simulink model "Verification_Component_Primitive_replacement"  (R2012b)
settings: Solver=FixedStepDiscrete  StartTime=0.0  StopTime=10.0  FixedStep=0.1  RelTol=1e-3
libraries: sldvlib x15, simulink x1
settings Model: sldv_blockreplacement_configurable_lib=Verification_Component_Primitive_rt_lib  Creator=Kerianne  LastModifiedBy=Kerianne
settings DataIOCC: SaveFormat=Structure
settings OptimizationCC: InlineParams=on
settings DebuggingCC: ArtificialAlgebraicLoopMsg=none

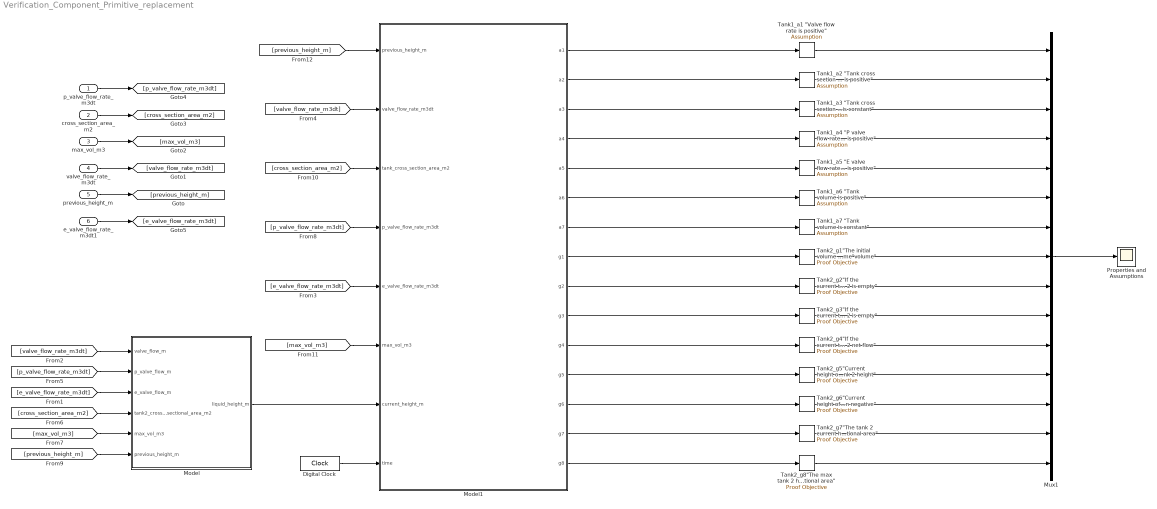
== system Verification_Component_Primitive_replacement ==
  p_valve_flow_rate_m3dt : Inport  OutDataTypeStr=double
  cross_section_area_m2 : Inport  Port=2  OutDataTypeStr=double
  max_vol_m3 : Inport  Port=3  OutDataTypeStr=double
  valve_flow_rate_m3dt : Inport  Port=4  OutDataTypeStr=double
  previous_height_m : Inport  Port=5  OutDataTypeStr=double
  e_valve_flow_rate_m3dt1 : Inport  Port=6  OutDataTypeStr=double
  Digital Clock : DigitalClock  SampleTime=0.1
  Model : Subsystem  TreatAsAtomicUnit=on  mask(Sldv ModelReference(Model name:Tank2_Primitives) Replacement){ModelName=Tank2_Primitives, ParameterArgumentNames=, ParameterArgumentValues=, SimulationMode=Normal}
      mask help: Replacement for the Model Reference block that references the model Tank2_Primitives. If Model arguments are specified on the Model Reference block, then they will appear in the mask parameters.
  Model1 : Subsystem  TreatAsAtomicUnit=on  mask(Sldv ModelReference(Model name:Properties_Tank2_Primitives) Replacement){ModelName=Properties_Tank2_Primitives, ParameterArgumentNames=, ParameterArgumentValues=, SimulationMode=Normal}
      mask help: Replacement for the Model Reference block that references the model Properties_Tank2_Primitives. If Model arguments are specified on the Model Reference block, then they will appear in the mask parameters.
  Mux1 : Mux  Inputs=15
  Properties and Assumptions : Scope
      settings: ShowLegends=on
  "Tank1_a1 \"Valve flow rate is positive\"" : sldvlib/Objectives and Constraints/Assumption  enabled=on  customAVTBlockType=Assumption  intervals=true  initial=off  dispValues=on  outEnabled=on
      settings: AttributesFormatString=%<intervals>
  "Tank1_a2 \"Tank cross section area is positive\"" : sldvlib/Objectives and Constraints/Assumption  enabled=on  customAVTBlockType=Assumption  intervals=true  initial=off  dispValues=on  outEnabled=on
      settings: AttributesFormatString=%<intervals>
  "Tank1_a3 \"Tank cross section area is constant\"" : sldvlib/Objectives and Constraints/Assumption  enabled=on  customAVTBlockType=Assumption  intervals=true  initial=off  dispValues=on  outEnabled=on
      settings: AttributesFormatString=%<intervals>
  "Tank1_a4 \"P valve flow rate is positive\"" : sldvlib/Objectives and Constraints/Assumption  enabled=on  customAVTBlockType=Assumption  intervals=true  initial=off  dispValues=on  outEnabled=on
      settings: AttributesFormatString=%<intervals>
  "Tank1_a5 \"E valve flow rate is positive\"" : sldvlib/Objectives and Constraints/Assumption  enabled=on  customAVTBlockType=Assumption  intervals=true  initial=off  dispValues=on  outEnabled=on
      settings: AttributesFormatString=%<intervals>
  "Tank1_a6 \"Tank volume is positive\"" : sldvlib/Objectives and Constraints/Assumption  enabled=on  customAVTBlockType=Assumption  intervals=true  initial=off  dispValues=on  outEnabled=on
      settings: AttributesFormatString=%<intervals>
  "Tank1_a7 \"Tank volume is constant\"" : sldvlib/Objectives and Constraints/Assumption  enabled=on  customAVTBlockType=Assumption  intervals=true  initial=off  dispValues=on  outEnabled=on
      settings: AttributesFormatString=%<intervals>
  "Tank2_g1\"The initial volume of tank 2 should be equivalent to the specified initial tank 2 volume\"volume\" " : sldvlib/Objectives and Constraints/Proof Objective  enabled=on  customAVTBlockType=Proof Objective  intervals=true  dispValues=on  outEnabled=on  enableStopSim=off
      settings: AttributesFormatString=%<intervals>
  "Tank2_g2\"If the current tank 2 volume plus the tank 2 net flow is less than the tank 2 minimum volume then tank 2 is empty\" " : sldvlib/Objectives and Constraints/Proof Objective  enabled=on  customAVTBlockType=Proof Objective  intervals=true  dispValues=on  outEnabled=on  enableStopSim=off
      settings: AttributesFormatString=%<intervals>
  "Tank2_g3\"If the current tank 2 volume plus the tank 2 net flow is less than the tank 2 minimum volume then tank 2 is empty\"" : sldvlib/Objectives and Constraints/Proof Objective  enabled=on  customAVTBlockType=Proof Objective  intervals=true  dispValues=on  outEnabled=on  enableStopSim=off
      settings: AttributesFormatString=%<intervals>
  "Tank2_g4\"If the current tank 2 volume plus the tank 2 net flow is greater than empty and less than the tank 2 maximum volume then the tank 2 volume changes by the tank 2 net flow\"" : sldvlib/Objectives and Constraints/Proof Objective  enabled=on  customAVTBlockType=Proof Objective  intervals=true  dispValues=on  outEnabled=on  enableStopSim=off
      settings: AttributesFormatString=%<intervals>
  "Tank2_g5\"Current height of tank 2 is equal or less than the max tank 2 height\"" : sldvlib/Objectives and Constraints/Proof Objective  enabled=on  customAVTBlockType=Proof Objective  intervals=true  dispValues=on  outEnabled=on  enableStopSim=off
      settings: AttributesFormatString=%<intervals>
  "Tank2_g6\"Current height of tank 2 is non negative\"" : sldvlib/Objectives and Constraints/Proof Objective  enabled=on  customAVTBlockType=Proof Objective  intervals=true  dispValues=on  outEnabled=on  enableStopSim=off
      settings: AttributesFormatString=%<intervals>
  "Tank2_g7\"The tank 2 current height is equal to the tank 2 current volume divided by the tank 2 cross sectional area\" " : sldvlib/Objectives and Constraints/Proof Objective  enabled=on  customAVTBlockType=Proof Objective  intervals=true  dispValues=on  outEnabled=on  enableStopSim=off
      settings: AttributesFormatString=%<intervals>
  "Tank2_g8\"The max tank 2 height is equal to the max tank 2 volume divided by tank 2 cross sectional area\"" : sldvlib/Objectives and Constraints/Proof Objective  enabled=on  customAVTBlockType=Proof Objective  intervals=true  dispValues=on  outEnabled=on  enableStopSim=off
      settings: AttributesFormatString=%<intervals>
  wires:
  Model/1(liquid_height_m) -> Model1/7(current_height_m)
  Mux1/1 -> Properties and Assumptions/1
  previous_height_m/1 -> [previous_height_m]
  valve_flow_rate_m3dt/1 -> [valve_flow_rate_m3dt]
  max_vol_m3/1 -> [max_vol_m3]
  p_valve_flow_rate_m3dt/1 -> [p_valve_flow_rate_m3dt]
  cross_section_area_m2/1 -> [cross_section_area_m2]
  Digital Clock/1 -> Model1/8(time)
  e_valve_flow_rate_m3dt1/1 -> [e_valve_flow_rate_m3dt]
  [valve_flow_rate_m3dt] -> Model/1(valve_flow_m)
  [p_valve_flow_rate_m3dt] -> Model/2(p_valve_flow_m)
  [e_valve_flow_rate_m3dt] -> Model/3(e_valve_flow_m)
  [cross_section_area_m2] -> Model/4(tank2_cross_sectional_area_m2)
  [max_vol_m3] -> Model/5(max_vol_m3)
  [previous_height_m] -> Model/6(previous_height_m)
  [previous_height_m] -> Model1/1(previous_height_m)
  [valve_flow_rate_m3dt] -> Model1/2(valve_flow_rate_m3dt)
  [cross_section_area_m2] -> Model1/3(tank_cross_section_area_m2)
  [p_valve_flow_rate_m3dt] -> Model1/4(p_valve_flow_rate_m3dt)
  [e_valve_flow_rate_m3dt] -> Model1/5(e_valve_flow_rate_m3dt)
  [max_vol_m3] -> Model1/6(max_vol_m3)
  Model1/7(a7) -> "Tank1_a7 \"Tank volume is constant\""/1
  Model1/6(a6) -> "Tank1_a6 \"Tank volume is positive\""/1
  Model1/5(a5) -> "Tank1_a5 \"E valve flow rate is positive\""/1
  Model1/4(a4) -> "Tank1_a4 \"P valve flow rate is positive\""/1
  Model1/3(a3) -> "Tank1_a3 \"Tank cross section area is constant\""/1
  Model1/2(a2) -> "Tank1_a2 \"Tank cross section area is positive\""/1
  Model1/1(a1) -> "Tank1_a1 \"Valve flow rate is positive\""/1
  "Tank1_a1 \"Valve flow rate is positive\""/1 -> Mux1/1
  "Tank1_a2 \"Tank cross section area is positive\""/1 -> Mux1/2
  "Tank1_a3 \"Tank cross section area is constant\""/1 -> Mux1/3
  "Tank1_a4 \"P valve flow rate is positive\""/1 -> Mux1/4
  "Tank1_a5 \"E valve flow rate is positive\""/1 -> Mux1/5
  "Tank1_a6 \"Tank volume is positive\""/1 -> Mux1/6
  "Tank1_a7 \"Tank volume is constant\""/1 -> Mux1/7
  Model1/8(g1) -> "Tank2_g1\"The initial volume of tank 2 should be equivalent to the specified initial tank 2 volume\"volume\" "/1
  Model1/9(g2) -> "Tank2_g2\"If the current tank 2 volume plus the tank 2 net flow is less than the tank 2 minimum volume then tank 2 is empty\" "/1
  Model1/10(g3) -> "Tank2_g3\"If the current tank 2 volume plus the tank 2 net flow is less than the tank 2 minimum volume then tank 2 is empty\""/1
  Model1/11(g4) -> "Tank2_g4\"If the current tank 2 volume plus the tank 2 net flow is greater than empty and less than the tank 2 maximum volume then the tank 2 volume changes by the tank 2 net flow\""/1
  Model1/12(g5) -> "Tank2_g5\"Current height of tank 2 is equal or less than the max tank 2 height\""/1
  Model1/13(g6) -> "Tank2_g6\"Current height of tank 2 is non negative\""/1
  Model1/14(g7) -> "Tank2_g7\"The tank 2 current height is equal to the tank 2 current volume divided by the tank 2 cross sectional area\" "/1
  Model1/15(g8) -> "Tank2_g8\"The max tank 2 height is equal to the max tank 2 volume divided by tank 2 cross sectional area\""/1
  "Tank2_g1\"The initial volume of tank 2 should be equivalent to the specified initial tank 2 volume\"volume\" "/1 -> Mux1/8
  "Tank2_g2\"If the current tank 2 volume plus the tank 2 net flow is less than the tank 2 minimum volume then tank 2 is empty\" "/1 -> Mux1/9
  "Tank2_g3\"If the current tank 2 volume plus the tank 2 net flow is less than the tank 2 minimum volume then tank 2 is empty\""/1 -> Mux1/10
  "Tank2_g4\"If the current tank 2 volume plus the tank 2 net flow is greater than empty and less than the tank 2 maximum volume then the tank 2 volume changes by the tank 2 net flow\""/1 -> Mux1/11
  "Tank2_g5\"Current height of tank 2 is equal or less than the max tank 2 height\""/1 -> Mux1/12
  "Tank2_g6\"Current height of tank 2 is non negative\""/1 -> Mux1/13
  "Tank2_g7\"The tank 2 current height is equal to the tank 2 current volume divided by the tank 2 cross sectional area\" "/1 -> Mux1/14
  "Tank2_g8\"The max tank 2 height is equal to the max tank 2 volume divided by tank 2 cross sectional area\""/1 -> Mux1/15

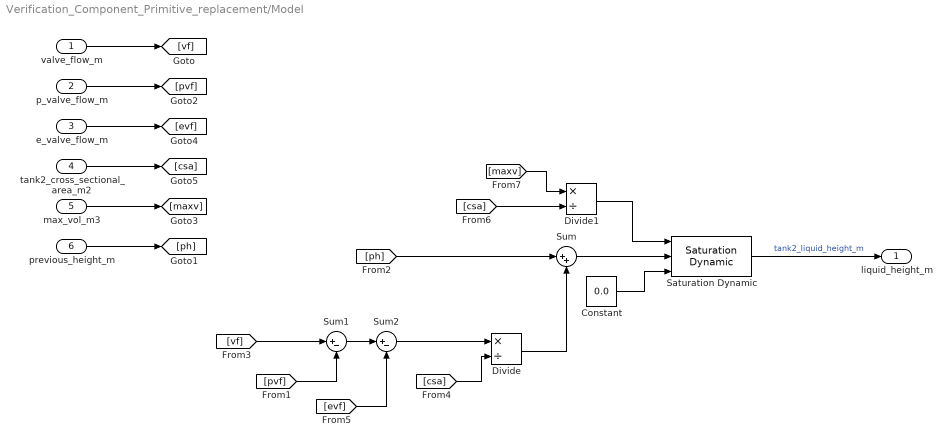
== system Verification_Component_Primitive_replacement/Model ==
  valve_flow_m : Inport  OutDataTypeStr=double  PortDimensions=1  SampleTime=[0.10000000000000001,0]
  p_valve_flow_m : Inport  Port=2  OutDataTypeStr=double  PortDimensions=1  SampleTime=[0.10000000000000001,0]
  e_valve_flow_m : Inport  Port=3  OutDataTypeStr=double  PortDimensions=1  SampleTime=[0.10000000000000001,0]
  tank2_cross_sectional_area_m2 : Inport  Port=4  OutDataTypeStr=double  PortDimensions=1  SampleTime=[0.10000000000000001,0]
  max_vol_m3 : Inport  Port=5  OutDataTypeStr=double  PortDimensions=1  SampleTime=[0.10000000000000001,0]
  previous_height_m : Inport  Port=6  OutDataTypeStr=double  PortDimensions=1  SampleTime=[0.10000000000000001,0]
  Constant : Constant  Value=0.0
  Divide : Product  Inputs=*/
  Divide1 : Product  Inputs=*/
  Saturation Dynamic : simulink/Discontinuities/Saturation Dynamic  OutMin=[]  OutMax=[]  OutDataTypeStr=Inherit: Same as second input  OutDataType=fixdt(1, 16)  OutScaling=2^-10  DoSatur=off
  Sum : Sum  Inputs=|++
  Sum1 : Sum  Inputs=|+-
  Sum2 : Sum  Inputs=|+-
  liquid_height_m : Outport  OutDataTypeStr=double  PortDimensions=1  SampleTime=[0.10000000000000001,0]
  wires:
  [evf] -> Sum2/2
  valve_flow_m/1 -> [vf]
  p_valve_flow_m/1 -> [pvf]
  Divide/1 -> Sum/2
  [csa] -> Divide/2
  [ph] -> Sum/1
  tank2_cross_sectional_area_m2/1 -> [csa]
  [vf] -> Sum1/1
  e_valve_flow_m/1 -> [evf]
  Sum2/1 -> Divide/1
  [pvf] -> Sum1/2
  Sum1/1 -> Sum2/1
  max_vol_m3/1 -> [maxv]
  Divide1/1 -> Saturation Dynamic/1
  Sum/1 -> Saturation Dynamic/2
  Constant/1 -> Saturation Dynamic/3
  [csa] -> Divide1/2
  [maxv] -> Divide1/1
  Saturation Dynamic/1 -> liquid_height_m/1  "tank2_liquid_height_m"
  previous_height_m/1 -> [ph]

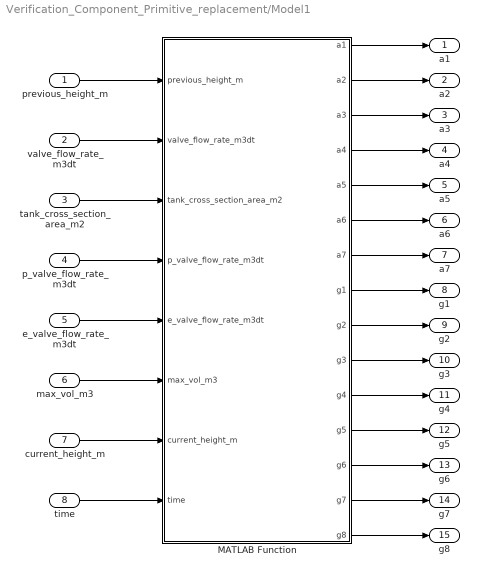
== system Verification_Component_Primitive_replacement/Model1 ==
  previous_height_m : Inport  OutDataTypeStr=double  PortDimensions=1  SampleTime=[0.10000000000000001,0]
  valve_flow_rate_m3dt : Inport  Port=2  OutDataTypeStr=double  PortDimensions=1  SampleTime=[0.10000000000000001,0]
  tank_cross_section_area_m2 : Inport  Port=3  OutDataTypeStr=double  PortDimensions=1  SampleTime=[0.10000000000000001,0]
  p_valve_flow_rate_m3dt : Inport  Port=4  OutDataTypeStr=double  PortDimensions=1  SampleTime=[0.10000000000000001,0]
  e_valve_flow_rate_m3dt : Inport  Port=5  OutDataTypeStr=double  PortDimensions=1  SampleTime=[0.10000000000000001,0]
  max_vol_m3 : Inport  Port=6  OutDataTypeStr=double  PortDimensions=1  SampleTime=[0.10000000000000001,0]
  current_height_m : Inport  Port=7  OutDataTypeStr=double  PortDimensions=1  SampleTime=[0.10000000000000001,0]
  time : Inport  Port=8  OutDataTypeStr=double  PortDimensions=1  SampleTime=[0.10000000000000001,0]
  MATLAB Function : MATLAB Function  TreatAsAtomicUnit=on
  a1 : Outport  OutDataTypeStr=boolean  PortDimensions=1  SampleTime=[0.10000000000000001,0]
  a2 : Outport  Port=2  OutDataTypeStr=boolean  PortDimensions=1  SampleTime=[0.10000000000000001,0]
  a3 : Outport  Port=3  OutDataTypeStr=boolean  PortDimensions=1  SampleTime=[0.10000000000000001,0]
  a4 : Outport  Port=4  OutDataTypeStr=boolean  PortDimensions=1  SampleTime=[0.10000000000000001,0]
  a5 : Outport  Port=5  OutDataTypeStr=boolean  PortDimensions=1  SampleTime=[0.10000000000000001,0]
  a6 : Outport  Port=6  OutDataTypeStr=boolean  PortDimensions=1  SampleTime=[0.10000000000000001,0]
  a7 : Outport  Port=7  OutDataTypeStr=boolean  PortDimensions=1  SampleTime=[0.10000000000000001,0]
  g1 : Outport  Port=8  OutDataTypeStr=boolean  PortDimensions=1  SampleTime=[0.10000000000000001,0]
  g2 : Outport  Port=9  OutDataTypeStr=boolean  PortDimensions=1  SampleTime=[0.10000000000000001,0]
  g3 : Outport  Port=10  OutDataTypeStr=boolean  PortDimensions=1  SampleTime=[0.10000000000000001,0]
  g4 : Outport  Port=11  OutDataTypeStr=boolean  PortDimensions=1  SampleTime=[0.10000000000000001,0]
  g5 : Outport  Port=12  OutDataTypeStr=boolean  PortDimensions=1  SampleTime=[0.10000000000000001,0]
  g6 : Outport  Port=13  OutDataTypeStr=boolean  PortDimensions=1  SampleTime=[0.10000000000000001,0]
  g7 : Outport  Port=14  OutDataTypeStr=boolean  PortDimensions=1  SampleTime=[0.10000000000000001,0]
  g8 : Outport  Port=15  OutDataTypeStr=boolean  PortDimensions=1  SampleTime=[0.10000000000000001,0]
  wires:
  MATLAB Function/15(g8) -> g8/1
  MATLAB Function/14(g7) -> g7/1
  MATLAB Function/13(g6) -> g6/1
  MATLAB Function/12(g5) -> g5/1
  MATLAB Function/11(g4) -> g4/1
  MATLAB Function/10(g3) -> g3/1
  MATLAB Function/9(g2) -> g2/1
  MATLAB Function/8(g1) -> g1/1
  MATLAB Function/7(a7) -> a7/1
  MATLAB Function/6(a6) -> a6/1
  MATLAB Function/5(a5) -> a5/1
  MATLAB Function/4(a4) -> a4/1
  MATLAB Function/3(a3) -> a3/1
  MATLAB Function/2(a2) -> a2/1
  MATLAB Function/1(a1) -> a1/1
  previous_height_m/1 -> MATLAB Function/1(previous_height_m)
  valve_flow_rate_m3dt/1 -> MATLAB Function/2(valve_flow_rate_m3dt)
  tank_cross_section_area_m2/1 -> MATLAB Function/3(tank_cross_section_area_m2)
  p_valve_flow_rate_m3dt/1 -> MATLAB Function/4(p_valve_flow_rate_m3dt)
  e_valve_flow_rate_m3dt/1 -> MATLAB Function/5(e_valve_flow_rate_m3dt)
  max_vol_m3/1 -> MATLAB Function/6(max_vol_m3)
  current_height_m/1 -> MATLAB Function/7(current_height_m)
  time/1 -> MATLAB Function/8(time)

== matlab function Verification_Component_Primitive_replacement/Model1/MATLAB Function ==
  data: a1 output; a2 output; a3 output; a4 output; a5 output; a6 output; a7 output; previous_height_m input; valve_flow_rate_m3dt input; tank_cross_section_area_m2 input; p_valve_flow_rate_m3dt input; e_valve_flow_rate_m3dt input; max_vol_m3 input; g1 output; current_height_m input; time input; g2 output; g3 output; g4 output; g5 output; g6 output; g7 output; g8 output
function [a1, a2, a3, a4, a5, a6, a7, g1, g2, g3, g4, g5, g6, g7, g8]   = verification_condition(previous_height_m, valve_flow_rate_m3dt, tank_cross_section_area_m2, p_valve_flow_rate_m3dt, e_valve_flow_rate_m3dt, max_vol_m3, current_height_m, time)

% Updated 27 Feb 2015 from 20150205 tank2.aadl

persistent pre_max_vol_m3
if isempty(pre_max_vol_m3)
    pre_max_vol_m3 = max_vol_m3;
end
persistent pre_tank_cross_section_area_m2
if isempty(pre_tank_cross_section_area_m2)
    pre_tank_cross_section_area_m2 = tank_cross_section_area_m2;
end

tank_height_m = max_vol_m3/tank_cross_section_area_m2;
current_volume_m3 = current_height_m*tank_cross_section_area_m2;
previous_volume_m3 = previous_height_m*tank_cross_section_area_m2;
net_flow_m3dt = valve_flow_rate_m3dt-p_valve_flow_rate_m3dt-e_valve_flow_rate_m3dt;
initial_height_m = 0.0;

% Assumptions
% assume "Valve flow rate is positive"
a1 = valve_flow_rate_m3dt >= 0.0;
% assume "Tank cross section area is positive"
a2 = tank_cross_section_area_m2 >= 0.0;
% assume "Tank cross section area is constant"
a3 = pre_tank_cross_section_area_m2 == tank_cross_section_area_m2;
% assume "P valve flow rate is positive"
a4 = p_valve_flow_rate_m3dt >= 0.0;
% assume "E valve flow rate is positive"
a5 = e_valve_flow_rate_m3dt >= 0.0;
% assume "Tank volume is positive"
a6 = max_vol_m3 >= 0;
% assume "Tank volume is constant"
a7 = pre_max_vol_m3 == max_vol_m3;
% previous hight - taken out


			
% guarantee "The initial volume of tank 2 should be equivalent to the specified initial tank 2 volume"
g1 = initially_empty(initial_height_m, previous_height_m,time,tank_cross_section_area_m2);
% guarantee "If the current tank 2 volume plus the tank 2 net flow is greater than the tank 2 maximum volume then tank 2 is full"
g2 = full_cond(current_volume_m3, net_flow_m3dt, max_vol_m3);	
% guarantee "If the current tank 2 volume plus the tank 2 net flow is less than the tank 2 minimum volume then tank 2 is empty" 
g3 = empty_cond(current_volume_m3, net_flow_m3dt);
% guarantee "If the current tank 2 volume plus the tank 2 net flow is greater than empty and less than the tank 2 maximum volume then the tank 2 volume changes by the tank 2 net flow"
g4 = tank_volume_update(current_volume_m3, net_flow_m3dt, max_vol_m3, previous_volume_m3);
% guarantee "Current height of tank 2 is equal or less than the max tank 2 height" 
g5 = tank_less_or_equal_full(current_height_m, tank_height_m);
% guarantee "Current height of tank 2 is non negative"
g6 = current_height_m >= 0.0;
% guarantee "The tank 2 current height is equal to the tank 2 current volume divided by the tank 2 cross sectional area" 
g7 = math_check(current_height_m, current_volume_m3, tank_cross_section_area_m2);
% guarantee "The max tank 2 height is equal to the max tank 2 volume divided by tank 2 cross sectional area"
g8 = math_check_2(tank_height_m, max_vol_m3, tank_cross_section_area_m2); 
% % guarantee "The current tank 2 height is the current tank 2 volume divided by the tank 2 cross sectional area"
% g9 = math_check_3(current_height_m, current_volume_m3, tank_cross_section_area_m2);
% % guarantee "The output height of tank 2 should equal the calculated height of tank 2"
% g10 = math_check_4(current_height_m, p_valve_flow_rate_m3dt, e_valve_flow_rate_m3dt, valve_flow_rate_m3dt, tank_cross_section_area_m2, previous_height_m);

function c = implies(a,b)      
     c = ((not (a)) || b);
% g1 "The initial volume of tank 2 should be equivalent to the specified initial tank 2 volume"
function result = initially_empty(initial_height_m, previous_height_m, time, tank_cross_section_area_m2)
    UnderThisCondition = (time == 0.0);
    ResultShouldBe = (previous_height_m*tank_cross_section_area_m2 == initial_height_m*tank_cross_section_area_m2);
    result = implies(UnderThisCondition, ResultShouldBe);
% g2 "If the current tank 2 volume plus the tank 2 net flow is greater than the tank 2 maximum volume then tank 2 is full"
function result = full_cond(current_volume_m3, net_flow_m3dt, tank_volume_m3)
    UnderThisCondition = (current_volume_m3 + net_flow_m3dt >= tank_volume_m3);
    ResultShouldBe = (current_volume_m3 == tank_volume_m3);
    result = implies(UnderThisCondition, ResultShouldBe);
% g3 "If the current tank 2 volume plus the tank 2 net flow is less than the tank 2 minimum volume then tank 2 is empty" 
function result = empty_cond(current_volume_m3, net_flow_m3dt)    
    UnderThisCondition = (current_volume_m3 + net_flow_m3dt <= 0.0);
    ResultShouldBe = (current_volume_m3 == 0.0);
    result = implies(UnderThisCondition, ResultShouldBe);
% g4 "If the current tank 2 volume plus the tank 2 net flow is greater than empty and less than the tank 2 maximum volume then the tank 2 volume changes by the tank 2 net flow"
function result = tank_volume_update(current_volume_m3, net_flow_m3dt, tank_volume_m3, previous_volume_m3)   
    UnderThisCondition = ((current_volume_m3 + net_flow_m3dt <= tank_volume_m3) && (current_volume_m3 + net_flow_m3dt >= 0.0));
    ResultShouldBe = (current_volume_m3 == previous_volume_m3 + net_flow_m3dt);
    result = implies(UnderThisCondition, ResultShouldBe);
% g5 "Current height of tank 2 is equal or less than the max tank 2 height"
function result = tank_less_or_equal_full(current_height_m, tank_height_m)   
    result = (current_height_m <= tank_height_m);
% g6 "Current height of tank 2 is non negative"
function result = tank_height_not_negative(current_height_m)   
    result = (current_height_m >= 0);
% g7 "The tank 2 current height is equal to the tank 2 current volume divided by the tank 2 cross sectional area" 
function result =  math_check(current_height_m, current_volume_m3, tank_cross_section_area_m2)
    result = (current_height_m == current_volume_m3 / tank_cross_section_area_m2);
% g8 "The max tank 2 height is equal to the max tank 2 volume divided by tank 2 cross sectional area"
function result =  math_check_2(tank_height_m, tank_volume_m3, tank_cross_section_area_m2)
    result = (tank_height_m == tank_volume_m3/ tank_cross_section_area_m2);
% g9 "The current tank 2 height is the current tank 2 volume divided by the tank 2 cross sectional area"
function result = math_check_3(current_height_m, current_volume_m3, tank_cross_section_area_m2)
 	result = (current_height_m == current_volume_m3 / tank_cross_section_area_m2);
% g10 "The output height of tank 2 should equal the calculated height of tank 2"
function result = math_check_4(current_height_m, p_valve_flow_rate_m3dt, e_valve_flow_rate_m3dt, valve_flow_rate_m3dt, tank_cross_section_area_m2, previous_height_m)
    result = (current_height_m == ((valve_flow_rate_m3dt-p_valve_flow_rate_m3dt-e_valve_flow_rate_m3dt)/tank_cross_section_area_m2) +previous_height_m);
